simulink model "Flatten2_export_export"  (Simulink 7.9)
settings: Solver=ode45  StartTime=0.0  StopTime=10.0  RelTol=1e-3
settings Model: Creator=boakes  LastModifiedBy=boakes

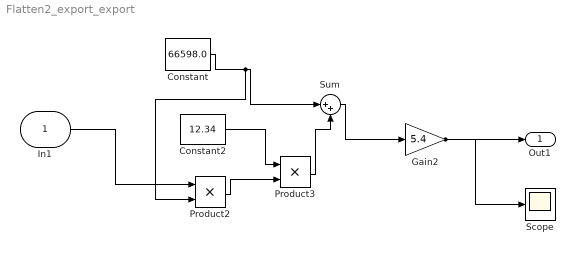
== system Flatten2_export_export ==
  In1 : Inport
  Constant : Constant  Value=66598.0
  Constant2 : Constant  Value=12.34
  Gain2 : Gain  Gain=5.4
  Product2 : Product  RndMeth=Zero
  Product3 : Product  RndMeth=Zero
  Scope : Scope
      settings: SaveName=ScopeData2
  Sum : Sum  Inputs=|++
  Out1 : Outport
  wires:
  Gain2/1 -> Scope/1, Out1/1
  Constant/1 -> Sum/1, Product2/2
  In1/1 -> Product2/1
  Product3/1 -> Sum/2
  Product2/1 -> Product3/2
  Sum/1 -> Gain2/1
  Constant2/1 -> Product3/1
